simulink model "Brain_Insulin32"  (R2018a)
settings: Solver=VariableStepAuto  StartTime=0.0  StopTime=10.0  RelTol=1e-3
undefined symbols (not defined in the file): Q_i_B, V_i_B
settings Model: Creator=cgonterman  LastModifiedBy=cgonterman

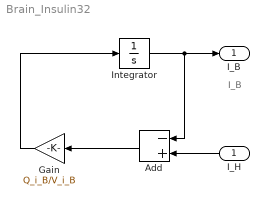
== system Brain_Insulin32 ==
  note: I_B
  I_H : Inport
  Add : Sum  Inputs=-+
  Gain : Gain  Gain=Q_i_B/V_i_B
  Integrator : Integrator
  "I_B " : Outport
  wires:
  I_H/1 -> Add/2
  Integrator/1 -> Add/1, "I_B "/1
  Add/1 -> Gain/1
  Gain/1 -> Integrator/1
